simulink model "DCDCSmlnk"  (Simulink 7.7)
settings: Solver=ode45  StartTime=0.0  StopTime=30  RelTol=1e-6
values from neighbouring files (symbols this model uses):
  A1 = DCDC_cont.A{1}    [dc-dc_converter.m]
  A2 = DCDC_cont.A{2}    [dc-dc_converter.m]
  B1 = DCDC_cont.B{1}    [dc-dc_converter.m]
  DCDCController_name = 'DCDCController'    [dc-dc_converter.m]
  uini = [1;1]    [dc-dc_converter.m]
  xini = [1.35;5.65]    [dc-dc_converter.m]
settings Model: Creator=manuelmazo  LastModifiedBy=manuelmazo  ExtModeAutoUpdateStatusClock=off
settings OptimizationCC: InitFltsAndDblsToZero=on
settings DebuggingCC: SaveWithParameterizedLinksMsg=none  StrictBusMsg=Warning
settings SFSimCC: SimParseCustomCode=off
settings GRTTargetCC: TargetFcnLib=ansi_tfl_tmw.mat

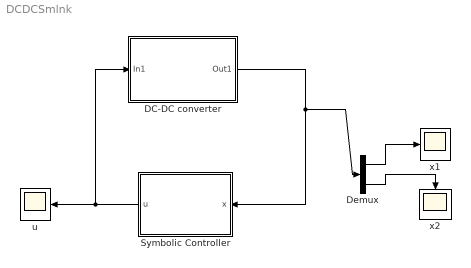
== system DCDCSmlnk ==
  DC-DC converter : Subsystem
  Demux : Demux  Outputs=2
  "Symbolic Controller " : Subsystem  mask{contr_name=DCDCController_name, uini=uini}
      mask prompts: contr_name "Controller Name"; uini "Initial Controller State"
      mask init:
      | load(strcat(contr_name,'_symb'), 'params_symb');
  u : Scope
      settings: SaveName=ScopeData3
  x1 : Scope
      settings: YMin=0.1  YMax=1.4
  x2 : Scope
      settings: YMin=5.5975  YMax=5.64  SaveName=ScopeData2
  wires:
  Demux/1 -> x1/1
  Demux/2 -> x2/1
  "Symbolic Controller "/1(u) -> u/1, DC-DC converter/1(In1)
  DC-DC converter/1(Out1) -> "Symbolic Controller "/1(x), Demux/1

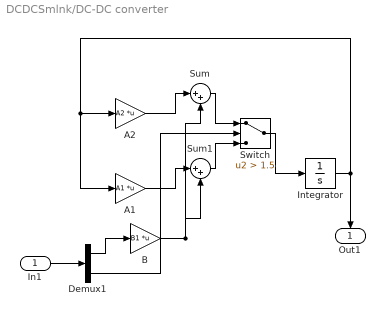
== system DCDCSmlnk/DC-DC converter ==
  In1 : Inport
  A1 : Gain  Gain=A1  Multiplication=Matrix(K*u)
  A2 : Gain  Gain=A2  Multiplication=Matrix(K*u)
  B : Gain  Gain=B1  Multiplication=Matrix(K*u)
  Demux1 : Demux  Outputs=2
  Integrator : Integrator  InitialCondition=xini
  Sum : Sum  Inputs=|++
  Sum1 : Sum  Inputs=|++
  Switch : Switch  Criteria=u2 > Threshold  Threshold=1.5
  Out1 : Outport
  wires:
  Integrator/1 -> A1/1, A2/1, Out1/1
  A1/1 -> Sum1/1
  A2/1 -> Sum/1
  B/1 -> Sum1/2, Sum/2
  Demux1/2 -> Switch/2
  Sum1/1 -> Switch/3
  Sum/1 -> Switch/1
  Switch/1 -> Integrator/1
  Demux1/1 -> B/1
  In1/1 -> Demux1/1

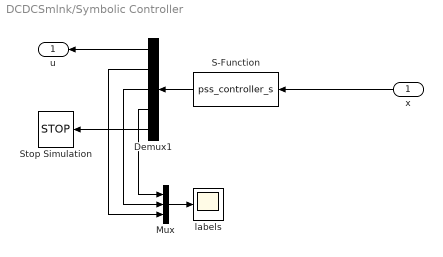
== system DCDCSmlnk/Symbolic Controller  ==
  x : Inport
  Demux1 : Demux  Outputs=5
  Mux : Mux  Inputs=3
  S-Function : S-Function  FunctionName=pss_controller_s  Parameters=params_symb, contr_name, uini  EnableBusSupport=off
  Stop Simulation : Stop
  labels : Scope
  u : Outport
  wires:
  S-Function/1 -> Demux1/1
  Demux1/4 -> Mux/1
  Demux1/3 -> Mux/2
  Demux1/2 -> Mux/3
  x/1 -> S-Function/1
  Demux1/1 -> u/1
  Demux1/5 -> Stop Simulation/1
  Mux/1 -> labels/1
